simulink model "system"  (R2019a)
settings: Solver=VariableStepAuto  StartTime=0.0  StopTime=15  RelTol=1e-3  AbsTol=1e-9
values from neighbouring files (symbols this model uses):
  A = pi*(r.^2)    [tank.m]
  g = 9.80665    [tank.m]
  h_d = 1.8    [tank.m]
  K = 1    [tank.m]
  R = 65360.93438    [tank.m]
  rho = 997    [tank.m]
settings Model: Creator=Luis Hernandez  LastModifiedBy=Luis Hernandez
settings DataIOCC: SaveOutput=off  SignalLogging=off  DSMLogging=off  SaveTime=off  ReturnWorkspaceOutputs=off

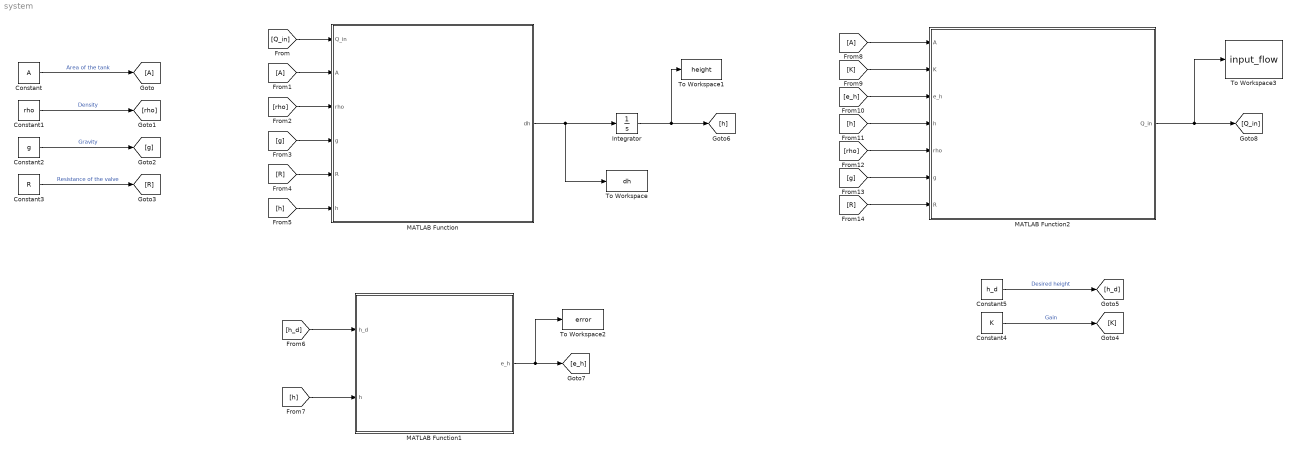
== system system ==
  Constant : Constant  Value=A
  Constant1 : Constant  Value=rho
  Constant2 : Constant  Value=g
  Constant3 : Constant  Value=R
  Constant4 : Constant  Value=K
  Constant5 : Constant  Value=h_d
  Integrator : Integrator
  MATLAB Function : MATLAB Function  TreatAsAtomicUnit=on
  MATLAB Function1 : MATLAB Function  TreatAsAtomicUnit=on
  MATLAB Function2 : MATLAB Function  TreatAsAtomicUnit=on
  To Workspace : ToWorkspace  VariableName=dh  SaveFormat=Timeseries  SampleTime=-1
  To Workspace1 : ToWorkspace  VariableName=height  SaveFormat=Timeseries  SampleTime=-1
  To Workspace2 : ToWorkspace  VariableName=error  SaveFormat=Timeseries  SampleTime=-1
  To Workspace3 : ToWorkspace  VariableName=input_flow  SaveFormat=Timeseries  SampleTime=-1
  wires:
  Constant/1 -> [A]  "Area of the tank"
  Constant1/1 -> [rho]  "Density"
  Constant2/1 -> [g]  "Gravity"
  Constant3/1 -> [R]  "Resistance of the valve"
  Constant4/1 -> [K]  "Gain"
  Constant5/1 -> [h_d]  "Desired height"
  [Q_in] -> MATLAB Function/1(Q_in)
  [A] -> MATLAB Function/2(A)
  [rho] -> MATLAB Function/3(rho)
  [g] -> MATLAB Function/4(g)
  [R] -> MATLAB Function/5(R)
  [h] -> MATLAB Function/6(h)
  MATLAB Function/1(dh) -> To Workspace/1, Integrator/1
  Integrator/1 -> To Workspace1/1, [h]
  [h_d] -> MATLAB Function1/1(h_d)
  [h] -> MATLAB Function1/2(h)
  MATLAB Function1/1(e_h) -> To Workspace2/1, [e_h]
  [A] -> MATLAB Function2/1(A)
  [K] -> MATLAB Function2/2(K)
  [e_h] -> MATLAB Function2/3(e_h)
  [h] -> MATLAB Function2/4(h)
  [rho] -> MATLAB Function2/5(rho)
  [g] -> MATLAB Function2/6(g)
  [R] -> MATLAB Function2/7(R)
  MATLAB Function2/1(Q_in) -> To Workspace3/1, [Q_in]

== matlab function system/MATLAB Function1 ==
  data: h_d input; e_h output; h input
function e_h = error(h_d, h)

% Error function
e_h = h_d - h;

== matlab function system/MATLAB Function ==
  data: Q_in input; dh output; A input; rho input; g input; R input; h input
function dh = system(Q_in, A, rho, g, R, h)

% Differential equation of the system
dh = (Q_in / A) - h * ((rho * g)/ (A * R));

== matlab function system/MATLAB Function2 ==
  data: A input; Q_in output; K input; e_h input; h input; rho input; g input; R input
function Q_in = control(A, K, e_h, h, rho, g, R)

% Control function
Q_in = A * K * e_h + (h * rho * g)/R;
